simulink model "sampleModel1969"  (R2023a)
settings: Solver=VariableStepAuto  StartTime=0.0  StopTime=10.0  RelTol=1e-3
libraries: hdlsllib x6, simulink x2
settings Model: Creator=user1  LastModifiedBy=user1

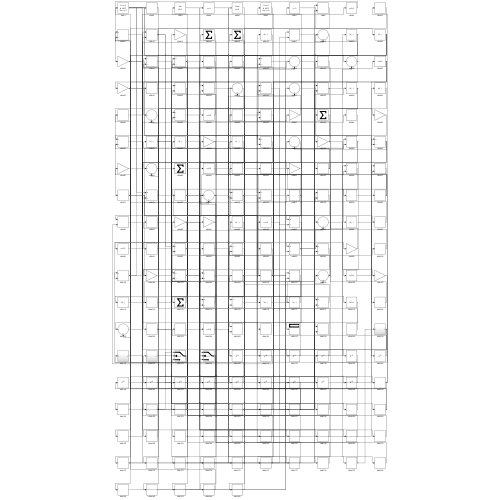
[thumbnail: Simulink's stored preview of the top-level diagram]
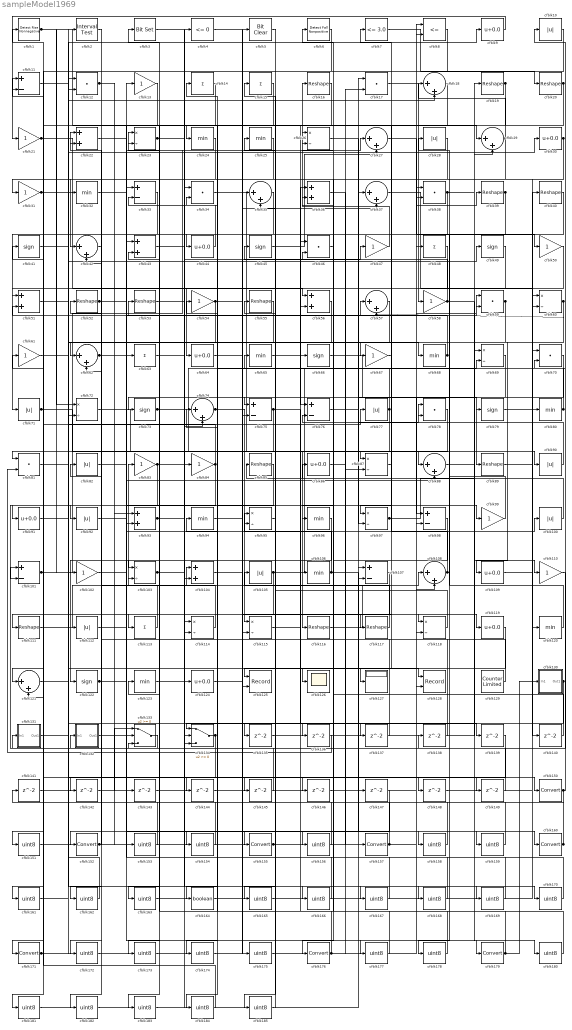
== system sampleModel1969 ==
  cfblk1 : hdlsllib/Logic and Bit Operations/Detect Rise Nonnegative  vinit=0  OutDataTypeStr=boolean
  cfblk{10,28,71,77,82,90,92,100,105,112} (10 alike) : Abs  SaturateOnIntegerOverflow=off
  cfblk{11,33,75..76,98,101,107} (7 alike) : Sum  Inputs=+-
  cfblk{13,21,31,47,50,54,58,61,67,83..84,99,102,110} (14 alike) : Gain
  cfblk{23,26,60,69,72,87,95,97,103,114..115,118} (12 alike) : Product  Inputs=*/  RndMeth=Zero  SaturateOnIntegerOverflow=on
  cfblk{22,36,43,51,56,93,104} (7 alike) : Sum
  cfblk{24..25,32,65,68,80,94,96,106,120,123} (11 alike) : MinMax
  cfblk{18,27,29,35,37,42,57,62,74,88,108,121} (12 alike) : Sum  Inputs=|++
  cfblk{9,30,44,64,86,91,109,119,124} (9 alike) : Bias  Bias=0.0  SaturateOnIntegerOverflow=off
  cfblk{16,19..20,39..40,52..53,55,85,89,111,116..117} (13 alike) : Reshape
  cfblk{14..15,48,63,113} (5 alike) : Sum  Inputs=+
  cfblk{12,17,34,38,46,59,70,78,81} (9 alike) : DotProduct  OutDataTypeStr=Inherit: Inherit via internal rule
  cfblk{41,45,49,66,73,79,122} (7 alike) : Signum
  cfblk125 : Record  FileSettingsInternal="{\"entries\":[{\"content\":{\"excelSettings\":{\"content\":{},\"type\":\"Streamout.ExcelSettings\"}},\"type\":\"Streamout.FileSettingStorage\",\"uuid\":\"\"}],\"packageUris\":[\"http:\\/\\/schema.mathworks.com\\/mf0\\/streamout_blocks\\/R2020a\"],\"version\":\"1.0\"}"  Layout=[1 1]  SignalsInternal="{\"entries\":[{\"content\":{\"signals\":[{\"content\":{\"blockPath\":[],\"dimensions\":[1],\"domain\":\"\",\"lineColor\":\"#a2142f\",\"plots\":[1],\"port\":1,\"signalID\":5545,\"signalName\":\"XY Graph:1\"},\"type\":\"RecordBlkView.Signal\",\"uuid\":\"\"},{\"content\":{\"blockPath\":[],\"dimensions\":[1],\"domain\":\"\",\"lineColor\":\"#139fff\",\"plots\":[1],\"port\":2,\"signalID\":5548,\"signalName\":\"XY Graph:2\"},\"type\":\"RecordBlkView.Signal\",\"uuid\":\"\"}]},\"type\":\"RecordBlkView.InputSignals\",\"uuid\":\"\"}],\"packageUris\":[\"http:\\/\\/schema.mathworks.com\\/mf0\\/streamout_blocks\\/R2020a\"],\"version\":\"1.0\"}"  VisualizationBindings="{\"xyplotplugin\":{\"info\":[{\"series\":[{\"bindingParametersList\":[{\"parameter\":\"X-Axis\",\"signalID\":5545,\"signalName\":\"XY Graph:1\"},{\"parameter\":\"Y-Axis\",\"signalID\":5548,\"signalName\":\"XY Graph:2\"}],\"seriesID\":49807}],\"subplotID\":1}]}}"  CompatibilityTag=XY  st=-1
  cfblk126 : Scope
  cfblk127 : Display
  cfblk128 : Record  FileSettingsInternal="{\"entries\":[{\"content\":{\"excelSettings\":{\"content\":{},\"type\":\"Streamout.ExcelSettings\"}},\"type\":\"Streamout.FileSettingStorage\",\"uuid\":\"\"}],\"packageUris\":[\"http:\\/\\/schema.mathworks.com\\/mf0\\/streamout_blocks\\/R2020a\"],\"version\":\"1.0\"}"  Layout=[1 1]  SignalsInternal="{\"entries\":[{\"content\":{\"signals\":[{\"content\":{\"blockPath\":[],\"dimensions\":[1],\"domain\":\"\",\"lineColor\":\"#a2142f\",\"plots\":[1],\"port\":1,\"signalID\":5553,\"signalName\":\"XY Graph:1\"},\"type\":\"RecordBlkView.Signal\",\"uuid\":\"\"},{\"content\":{\"blockPath\":[],\"dimensions\":[1],\"domain\":\"\",\"lineColor\":\"#139fff\",\"plots\":[1],\"port\":2,\"signalID\":5556,\"signalName\":\"XY Graph:2\"},\"type\":\"RecordBlkView.Signal\",\"uuid\":\"\"}]},\"type\":\"RecordBlkView.InputSignals\",\"uuid\":\"\"}],\"packageUris\":[\"http:\\/\\/schema.mathworks.com\\/mf0\\/streamout_blocks\\/R2020a\"],\"version\":\"1.0\"}"  VisualizationBindings="{\"xyplotplugin\":{\"info\":[{\"series\":[{\"bindingParametersList\":[{\"parameter\":\"X-Axis\",\"signalID\":5553,\"signalName\":\"XY Graph:1\"},{\"parameter\":\"Y-Axis\",\"signalID\":5556,\"signalName\":\"XY Graph:2\"}],\"seriesID\":38868}],\"subplotID\":1}]}}"  CompatibilityTag=XY  st=-1
  cfblk129 : hdlsllib/Sources/Counter Limited  uplimit=7  tsamp=-1
  cfblk130 : Subsystem
      settings: LibrarySourceBlock=|
      | hdlsllib/Ports &
      | Subsystems/Subsystem
  cfblk131 : Subsystem
      settings: LibrarySourceBlock=|
      | hdlsllib/Ports &
      | Subsystems/Subsystem
  cfblk132 : Subsystem
      settings: LibrarySourceBlock=|
      | hdlsllib/Ports &
      | Subsystems/Subsystem
  cfblk133 : Switch  SaturateOnIntegerOverflow=off  InputSameDT=off
  cfblk134 : Switch  SaturateOnIntegerOverflow=off  InputSameDT=off
  cfblk{135..149} (15 alike) : Delay  SampleTime=1
  cfblk{150,152,155,157,160,171,176,179} (8 alike) : DataTypeConversion  SaturateOnIntegerOverflow=off  RndMeth=Floor
  cfblk{151,153..154,156,158..159,161..163,165..170,172..175,177..178,180..185} (27 alike) : DataTypeConversion  OutDataTypeStr=uint8  SaturateOnIntegerOverflow=off  RndMeth=Floor
  cfblk164 : DataTypeConversion  OutDataTypeStr=boolean  SaturateOnIntegerOverflow=off  RndMeth=Floor
  cfblk2 : hdlsllib/Logic and Bit Operations/Interval Test  IntervalClosedRight=on  uplimit=0.5  IntervalClosedLeft=on  lowlimit=-0.5  OutDataTypeStr=boolean
  cfblk3 : simulink/Logic and Bit Operations/Bit Set  iBit=0
      settings: LibrarySourceBlock=|
      | hdlsllib/Logic and Bit
      | Operations/Bit Set
  cfblk4 : hdlsllib/Logic and Bit Operations/Compare To Zero  relop=<=  OutDataTypeStr=boolean
  cfblk5 : simulink/Logic and Bit Operations/Bit Clear  iBit=0
      settings: LibrarySourceBlock=|
      | hdlsllib/Logic and Bit
      | Operations/Bit Clear
  cfblk6 : hdlsllib/Logic and Bit Operations/Detect Fall Nonpositive  vinit=0  OutDataTypeStr=boolean
  cfblk7 : hdlsllib/Logic and Bit Operations/Compare To Constant  relop=<=  const=3.0  OutDataTypeStr=boolean
  cfblk8 : RelationalOperator  Operator=<=  OutDataTypeStr=boolean  InputSameDT=off
  wires:
  cfblk33/1 -> cfblk152/1
  cfblk49/1 -> cfblk64/1
  cfblk101/1 -> cfblk27/1, cfblk2/1
  cfblk16/1 -> cfblk24/1
  cfblk34/1 -> cfblk88/1
  cfblk74/1 -> cfblk119/1, cfblk134/1
  cfblk42/1 -> cfblk92/1
  cfblk79/1 -> cfblk80/1
  cfblk83/1 -> cfblk91/1, cfblk148/1, cfblk167/1
  cfblk17/1 -> cfblk58/1
  cfblk65/1 -> cfblk66/1
  cfblk93/1 -> cfblk163/1, cfblk170/1
  cfblk92/1 -> cfblk13/1
  cfblk114/1 -> cfblk83/1
  cfblk37/1 -> cfblk120/1
  cfblk40/1 -> cfblk71/1
  cfblk53/1 -> cfblk124/1
  cfblk24/1 -> cfblk81/1
  cfblk111/1 -> cfblk108/1
  cfblk3/1 -> cfblk34/1
  cfblk59/1 -> cfblk85/1, cfblk114/2
  cfblk47/1 -> cfblk16/1
  cfblk36/1 -> cfblk157/1
  cfblk78/1 -> cfblk113/1
  cfblk73/1 -> cfblk116/1, cfblk8/2
  cfblk56/1 -> cfblk62/1
  cfblk62/1 -> cfblk22/1, cfblk102/1, cfblk63/1
  cfblk91/1 -> cfblk77/1
  cfblk113/1 -> cfblk82/1
  cfblk70/1 -> cfblk89/1
  cfblk82/1 -> cfblk99/1
  cfblk29/1 -> cfblk31/1, cfblk18/1
  cfblk108/1 -> cfblk57/1, cfblk78/1
  cfblk120/1 -> cfblk65/1
  cfblk20/1 -> cfblk127/1, cfblk73/1, cfblk93/2, cfblk121/1
  cfblk133/1 -> cfblk131/1(In1)
  cfblk105/1 -> cfblk37/1, cfblk133/2
  cfblk75/1 -> cfblk111/1, cfblk137/1
  cfblk6/1 -> cfblk125/1
  cfblk32/1 -> cfblk160/1
  cfblk97/1 -> cfblk69/1, cfblk59/2
  cfblk19/1 -> cfblk87/1, cfblk115/1
  cfblk96/1 -> cfblk122/1
  cfblk10/1 -> cfblk51/1
  cfblk122/1 -> cfblk104/1, cfblk26/2
  cfblk11/1 -> cfblk112/1
  cfblk112/1 -> cfblk100/1
  cfblk15/1 -> cfblk44/1
  cfblk103/1 -> cfblk47/1, cfblk128/1
  cfblk68/1 -> cfblk51/2, cfblk53/1
  cfblk77/1 -> cfblk14/1, cfblk174/1
  cfblk84/1 -> cfblk101/2, cfblk11/1
  cfblk26/1 -> cfblk90/1
  cfblk81/1 -> cfblk30/1
  cfblk64/1 -> cfblk37/2
  cfblk45/1 -> cfblk27/2
  cfblk100/1 -> cfblk86/1
  cfblk86/1 -> cfblk87/2
  cfblk21/1 -> cfblk56/1, cfblk126/1
  cfblk99/1 -> cfblk28/1
  cfblk71/1 -> cfblk106/1, cfblk11/2, cfblk97/2
  cfblk31/1 -> cfblk76/1, cfblk18/2
  cfblk67/1 -> cfblk7/1
  cfblk66/1 -> cfblk98/1
  cfblk60/1 -> cfblk109/1, cfblk57/2, cfblk97/1
  cfblk2/1 -> cfblk62/2
  cfblk106/1 -> cfblk25/1, cfblk78/2, cfblk158/1
  cfblk115/1 -> cfblk69/2
  cfblk46/1 -> cfblk176/1
  cfblk25/1 -> cfblk42/1
  cfblk1/1 -> cfblk29/1, cfblk56/2, cfblk72/1, cfblk168/1
  cfblk121/1 -> cfblk49/1
  cfblk38/1 -> cfblk19/1, cfblk154/1
  cfblk58/1 -> cfblk45/1, cfblk110/1
  cfblk23/1 -> cfblk103/1, cfblk74/2
  cfblk48/1 -> cfblk171/1
  cfblk12/1 -> cfblk93/1, cfblk143/1
  cfblk9/1 -> cfblk21/1
  cfblk90/1 -> cfblk6/1
  cfblk117/1 -> cfblk95/1
  cfblk50/1 -> cfblk75/1
  cfblk134/1 -> cfblk151/1, cfblk172/1
  cfblk116/1 -> cfblk39/1
  cfblk57/1 -> cfblk125/2
  cfblk102/1 -> cfblk59/1
  cfblk132/1(Out1) -> cfblk155/1
  cfblk94/1 -> cfblk179/1
  cfblk72/1 -> cfblk114/1
  cfblk80/1 -> cfblk15/1, cfblk54/1
  cfblk129/1 -> cfblk26/1
  cfblk104/1 -> cfblk118/1
  cfblk7/1 -> cfblk20/1
  cfblk4/1 -> cfblk150/1
  cfblk41/1 -> cfblk9/1
  cfblk54/1 -> cfblk67/1, cfblk72/2
  cfblk130/1(Out1) -> cfblk144/1, cfblk145/1
  cfblk118/1 -> cfblk95/2
  cfblk61/1 -> cfblk68/1
  cfblk39/1 -> cfblk42/2, cfblk178/1
  cfblk14/1 -> cfblk104/2
  cfblk27/1 -> cfblk50/1
  cfblk76/1 -> cfblk79/1
  cfblk87/1 -> cfblk117/1
  cfblk52/1 -> cfblk88/2, cfblk177/1
  cfblk18/1 -> cfblk75/2
  cfblk30/1 -> cfblk96/1, cfblk60/2, cfblk134/3
  cfblk44/1 -> cfblk23/1
  cfblk109/1 -> cfblk40/1
  cfblk95/1 -> cfblk135/1
  cfblk135/1 -> cfblk29/2
  cfblk28/1 -> cfblk136/1
  cfblk136/1 -> cfblk81/2
  cfblk137/1 -> cfblk23/2
  cfblk110/1 -> cfblk138/1
  cfblk138/1 -> cfblk22/2
  cfblk51/1 -> cfblk139/1
  cfblk89/1 -> cfblk140/1
  cfblk140/1 -> cfblk76/2
  cfblk141/1 -> cfblk115/2
  cfblk8/1 -> cfblk142/1
  cfblk143/1 -> cfblk103/2
  cfblk144/1 -> cfblk98/2
  cfblk145/1 -> cfblk1/1
  cfblk131/1(Out1) -> cfblk146/1
  cfblk146/1 -> cfblk38/1
  cfblk148/1 -> cfblk60/1
  cfblk63/1 -> cfblk149/1
  cfblk149/1 -> cfblk101/1
  cfblk150/1 -> cfblk141/1, cfblk10/1, cfblk70/2
  cfblk151/1 -> cfblk4/1
  cfblk152/1 -> cfblk118/2, cfblk133/1, cfblk52/1
  cfblk22/1 -> cfblk153/1
  cfblk153/1 -> cfblk33/1
  cfblk154/1 -> cfblk33/2
  cfblk155/1 -> cfblk128/2, cfblk38/2
  cfblk98/1 -> cfblk156/1
  cfblk156/1 -> cfblk132/1(In1)
  cfblk157/1 -> cfblk134/2, cfblk121/2, cfblk108/2
  cfblk158/1 -> cfblk36/1
  cfblk142/1 -> cfblk159/1
  cfblk159/1 -> cfblk36/2
  cfblk160/1 -> cfblk41/1, cfblk105/1
  cfblk13/1 -> cfblk161/1
  cfblk161/1 -> cfblk32/1
  cfblk147/1 -> cfblk162/1
  cfblk162/1 -> cfblk12/1
  cfblk163/1 -> cfblk147/1
  cfblk85/1 -> cfblk164/1
  cfblk164/1 -> cfblk5/1
  cfblk5/1 -> cfblk165/1
  cfblk165/1 -> cfblk70/1
  cfblk43/1 -> cfblk166/1
  cfblk166/1 -> cfblk3/1
  cfblk167/1 -> cfblk43/1
  cfblk168/1 -> cfblk43/2
  cfblk123/1 -> cfblk169/1
  cfblk169/1 -> cfblk34/2
  cfblk170/1 -> cfblk123/1
  cfblk171/1 -> cfblk12/2, cfblk8/1
  cfblk172/1 -> cfblk48/1
  cfblk35/1 -> cfblk173/1
  cfblk173/1 -> cfblk17/1
  cfblk174/1 -> cfblk35/1
  cfblk124/1 -> cfblk175/1
  cfblk175/1 -> cfblk35/2
  cfblk176/1 -> cfblk74/1, cfblk17/2
  cfblk177/1 -> cfblk46/1
  cfblk178/1 -> cfblk46/2
  cfblk179/1 -> cfblk133/3, cfblk130/1(In1)
  cfblk88/1 -> cfblk180/1
  cfblk180/1 -> cfblk94/1
  cfblk107/1 -> cfblk181/1
  cfblk181/1 -> cfblk84/1
  cfblk139/1 -> cfblk182/1
  cfblk182/1 -> cfblk107/1
  cfblk69/1 -> cfblk183/1
  cfblk183/1 -> cfblk107/2
  cfblk55/1 -> cfblk184/1
  cfblk184/1 -> cfblk61/1
  cfblk119/1 -> cfblk185/1
  cfblk185/1 -> cfblk55/1

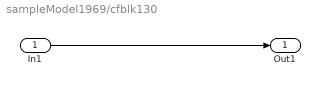
== system sampleModel1969/cfblk130 ==
  In1 : Inport
  Out1 : Outport
  wires:
  In1/1 -> Out1/1

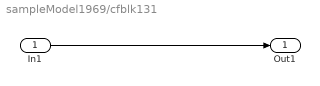
== system sampleModel1969/cfblk131 ==
  In1 : Inport
  Out1 : Outport
  wires:
  In1/1 -> Out1/1

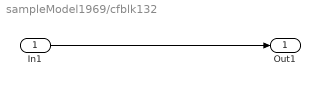
== system sampleModel1969/cfblk132 ==
  In1 : Inport
  Out1 : Outport
  wires:
  In1/1 -> Out1/1
